simulink model "simu_test4x2"  (Simulink 7.7)
settings: Solver=ode45  StartTime=0.0  StopTime=10.0  RelTol=1e-3
libraries: fuzblock x1
settings Model: Creator=Marcin  LastModifiedBy=Marcin

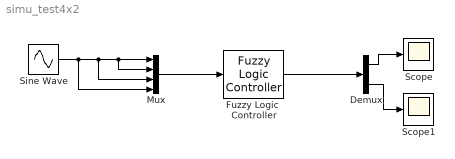
== system simu_test4x2 ==
  Demux : Demux  Outputs=2
  Fuzzy Logic  Controller : fuzblock/Fuzzy Logic  Controller  SystemSampleTime=-1  fis=fls
  Mux : Mux
  Scope : Scope
  Scope1 : Scope
  Sine Wave : Sin  SampleTime=0
  wires:
  Mux/1 -> Fuzzy Logic  Controller/1
  Fuzzy Logic  Controller/1 -> Demux/1
  Demux/1 -> Scope/1
  Demux/2 -> Scope1/1
  Sine Wave/1 -> Mux/1, Mux/2, Mux/3, Mux/4
